simulink model "pos_control2_test"  (R2016b)
settings: Solver=ode3  StartTime=0.0  StopTime=30  FixedStep=0.0025  RelTol=1e-3
model workspace: external: MATLAB File /home/hywel/Simulink/2017_10_drone/para_pos.m (data not in the file)
undefined symbols (not defined in the file or in its folder): bool_pos, control_mode, def, par, par_input, par_pos, position_setpoint, v_control_mode
(part 1 of 2)
settings Model: Creator=root  LastModifiedBy=root
settings OptimizationCC: DefaultParameterBehavior=Inlined
settings DebuggingCC: ParameterTunabilityLossMsg=error
settings HardwareCC: ProdBitPerLong=64  ProdHWDeviceType=Intel->x86-64 (Linux 64)
settings RTWCC: SystemTargetFile=ert.tlc  TemplateMakefile=ert_default_tmf  Description=Embedded Coder  GenerateReport=on  IncludeHyperlinkInReport=on  LaunchReport=on  GenerateTraceInfo=on  GenerateTraceReport=on  GenerateTraceReportSl=on  GenerateTraceReportSf=on  GenerateTraceReportEml=on
settings CodeAppCC: ForceParamTrailComments=on  IgnoreCustomStorageClasses=off  OperatorAnnotations=on  SimulinkDataObjDesc=on  SFDataObjDesc=on  MATLABFcnDesc=on  InsertBlockDesc=on  MATLABSourceComments=on
settings ERTTargetCC: TargetLangStandard=C99 (ISO)  GenerateSampleERTMain=on  InlinedParameterPlacement=NonHierarchical  ERTCustomFileTemplate=example_file_process.tlc

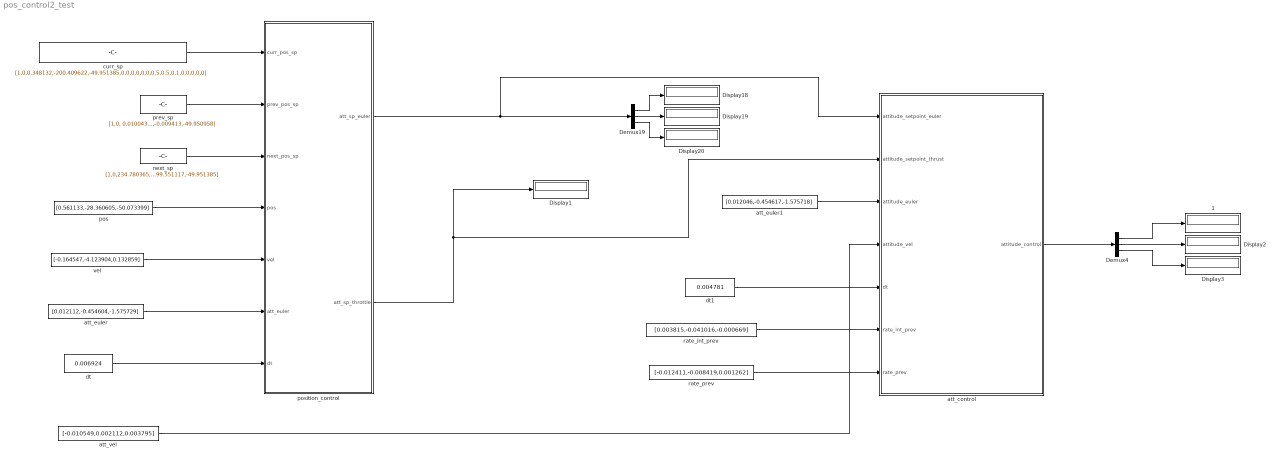
== system pos_control2_test ==
  1 : Display
  Demux19 : Demux  Outputs=3
  Demux4 : Demux  Outputs=3
  Display{1..3,18..20} (6 alike) : Display
  att_control : Subsystem
  att_euler : Constant  Value=[0.012112,-0.454604,-1.575729]
  att_euler1 : Constant  Value=[0.012046,-0.454617,-1.575718]
  att_vel : Constant  Value=[-0.010549,0.002112,0.003795]
  curr_sp : Constant  Value=[1,0,0.348132,-200.409622,-49.951385,0,0,0,0,0,0,0.5,0.5,0,1,0,0,0,0,0]
  dt : Constant  Value=0.006924
  dt1 : Constant  Value=0.004781
  next_sp : Constant  Value=[1,0,234.780365,-199.551117,-49.951385]
  pos : Constant  Value=[0.561133,-28.360605,-50.073399]
  position_control : Subsystem
  prev_sp : Constant  Value=[1,0, 0.010043,-0.009413,-49.950958]
  rate_int_prev : Constant  Value=[0.003815,-0.041016,-0.000669]
  rate_prev : Constant  Value=[-0.012411,-0.008419,0.001262]
  vel : Constant  Value=[-0.164547,-4.123904,0.132859]
  wires:
  pos/1 -> position_control/4(pos)
  vel/1 -> position_control/5(vel)
  curr_sp/1 -> position_control/1(curr_pos_sp)
  prev_sp/1 -> position_control/2(prev_pos_sp)
  next_sp/1 -> position_control/3(next_pos_sp)
  Demux19/2 -> Display19/1
  Demux19/3 -> Display20/1
  Demux19/1 -> Display18/1
  att_control/1(attitude_control) -> Demux4/1
  Demux4/2 -> Display2/1
  Demux4/1 -> 1/1
  Demux4/3 -> Display3/1
  att_euler/1 -> position_control/6(att_euler)
  att_vel/1 -> att_control/4(attitude_vel)
  dt/1 -> position_control/7(dt)
  rate_prev/1 -> att_control/7(rate_prev)
  rate_int_prev/1 -> att_control/6(rate_int_prev)
  dt1/1 -> att_control/5(dt)
  position_control/2(att_sp_throttle) -> att_control/2(attitude_setpoint_thrust), Display1/1
  position_control/1(att_sp_euler) -> att_control/1(attitude_setpoint_euler), Demux19/1
  att_euler1/1 -> att_control/3(attitude_euler)

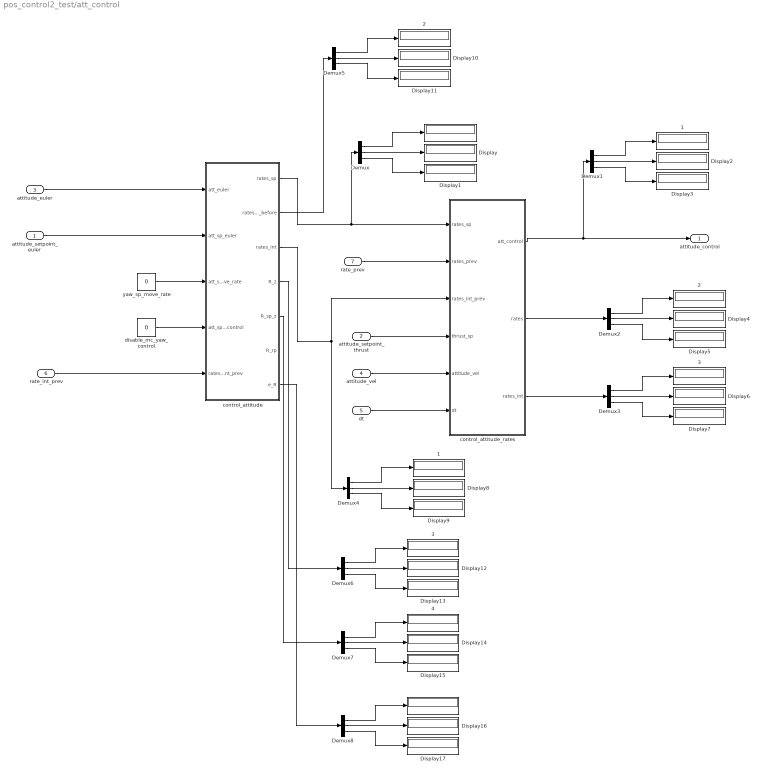
== system pos_control2_test/att_control ==
  attitude_setpoint_euler : Inport
  attitude_setpoint_thrust : Inport  Port=2
  attitude_euler : Inport  Port=3
  attitude_vel : Inport  Port=4
  dt : Inport  Port=5
  rate_int_prev : Inport  Port=6
  rate_prev : Inport  Port=7
   {,,1..4} (6 alike) : Display
  1 : Display
  2 : Display
  3 : Display
  Demux{,1..8} (9 alike) : Demux  Outputs=3
  Display{,1..17} (18 alike) : Display
  control_attitude : MATLAB Function  TreatAsAtomicUnit=on
  control_attitude_rates : MATLAB Function  TreatAsAtomicUnit=on
  disable_mc_yaw_control : Constant  Value=0
  yaw_sp_move_rate : Constant  Value=0
  attitude_control : Outport
  wires:
  yaw_sp_move_rate/1 -> control_attitude/3(att_sp_yaw_sp_move_rate)
  disable_mc_yaw_control/1 -> control_attitude/4(att_sp_disable_mc_yaw_control)
  control_attitude/1(rates_sp) -> Demux/1, control_attitude_rates/1(rates_sp)
  attitude_setpoint_euler/1 -> control_attitude/2(att_sp_euler)
  attitude_setpoint_thrust/1 -> control_attitude_rates/4(thrust_sp)
  attitude_euler/1 -> control_attitude/1(att_euler)
  attitude_vel/1 -> control_attitude_rates/5(attitude_vel)
  Demux/2 -> Display/1
  Demux/1 -> " "/1
  Demux/3 -> Display1/1
  control_attitude_rates/1(att_control) -> Demux1/1, attitude_control/1
  Demux1/2 -> Display2/1
  Demux1/1 -> 1/1
  Demux1/3 -> Display3/1
  control_attitude_rates/2(rates) -> Demux2/1
  Demux2/2 -> Display4/1
  Demux2/1 -> 2/1
  Demux2/3 -> Display5/1
  control_attitude_rates/3(rates_int) -> Demux3/1
  Demux3/2 -> Display6/1
  Demux3/1 -> 3/1
  Demux3/3 -> Display7/1
  dt/1 -> control_attitude_rates/6(dt)
  rate_int_prev/1 -> control_attitude/5(rates_int_prev)
  rate_prev/1 -> control_attitude_rates/2(rates_prev)
  control_attitude/3(rates_int) -> control_attitude_rates/3(rates_int_prev), Demux4/1
  Demux4/2 -> Display8/1
  Demux4/1 -> " 1"/1
  Demux4/3 -> Display9/1
  control_attitude/2(rates_sp_before) -> Demux5/1
  Demux5/2 -> Display10/1
  Demux5/1 -> " 2"/1
  Demux5/3 -> Display11/1
  control_attitude/4(R_z) -> Demux6/1
  Demux6/2 -> Display12/1
  Demux6/1 -> " 3"/1
  Demux6/3 -> Display13/1
  control_attitude/5(R_sp_z) -> Demux7/1
  Demux7/2 -> Display14/1
  Demux7/1 -> " 4"/1
  Demux7/3 -> Display15/1
  control_attitude/7(e_R) -> Demux8/1
  Demux8/2 -> Display16/1
  Demux8/1 -> " "/1
  Demux8/3 -> Display17/1

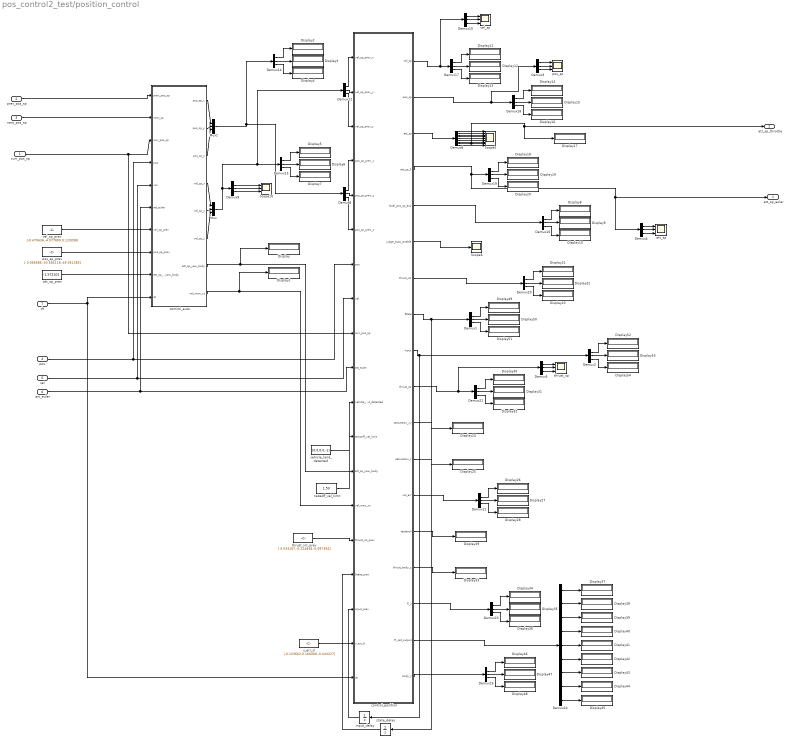
== system pos_control2_test/position_control ==
  curr_pos_sp : Inport
  prev_pos_sp : Inport  Port=2
  next_pos_sp : Inport  Port=3
  pos : Inport  Port=4
  vel : Inport  Port=5
  att_euler : Inport  Port=6
  dt : Inport  Port=7
  Demux{1..5,8..10,12,14..23,25} (20 alike) : Demux  Outputs=3
  Demux24 : Demux  Outputs=9
  Demux6 : Demux  Outputs=9
  Display{,1..54} (55 alike) : Display
  Mux : Mux  Inputs=3
  Mux1 : Mux  Inputs=3
  Scope10 : Scope  NumInputPorts=3
  Scope5 : Scope  NumInputPorts=9
  Scope6 : Scope
  att_sp : Scope  NumInputPorts=3
  att_sp_prev : Constant  Value=-1.572101
  control_auto : MATLAB Function  TreatAsAtomicUnit=on
  control_position : MATLAB Function  TreatAsAtomicUnit=on
  input_delay : UnitDelay  InitialCondition=[0,0,0]  SampleTime=-1
  pos_sp : Scope  NumInputPorts=3
  pos_sp_prev : Constant  Value=[ 0.066686,-33.584118,-49.951385]
  state_delay : UnitDelay  InitialCondition=[0,0,0]  SampleTime=-1
  takeoff_vel_limit : Constant  Value=1.53
  thrust_int_prev : Constant  Value=[ 0.034167,-0.224848,-0.087394]
  thrust_sp : Scope  NumInputPorts=3
  v_err_d : Constant  Value=[-0.123662,0.166068,-0.043227]
  vehicle_land_detected : Constant  Value=[0,0,0,0,-1]
  vel_sp : Scope  NumInputPorts=3
  vel_sp_prev : Constant  Value=[-0.470636,-4.977800,0.120098]
  att_sp_euler : Outport
  att_sp_throttle : Outport  Port=2
  wires:
  control_auto/7(att_sp_yaw_body) -> Display/1, control_position/13(att_sp_yaw_body)
  control_auto/8(vel_max_xy) -> Display1/1, control_position/14(vel_max_xy)
  takeoff_vel_limit/1 -> control_position/12(takeoff_vel_limit)
  vehicle_land_detected/1 -> control_position/11(vehicle_land_detected)
  next_pos_sp/1 -> control_auto/2(next_sp)
  prev_pos_sp/1 -> control_auto/1(prev_pos_sp)
  curr_pos_sp/1 -> control_auto/3(curr_pos_sp), control_position/9(curr_pos_sp)
  Demux6/1 -> Scope5/1
  Demux6/2 -> Scope5/2
  Demux6/3 -> Scope5/3
  control_position/3(att_sp) -> Demux6/1
  Demux6/4 -> Scope5/4
  Demux6/5 -> Scope5/5
  Demux6/6 -> Scope5/6
  Demux6/7 -> Scope5/7
  Demux6/9 -> Scope5/9
  control_position/5(local_pos_sp_acc) -> Demux16/1
  control_position/6(judge_auto_enable) -> Scope6/1
  Demux8/1 -> control_position/4(pos_sp_prev_x)
  Demux8/2 -> control_position/5(pos_sp_prev_y)
  Demux8/3 -> control_position/6(pos_sp_prev_z)
  Demux9/1 -> Scope10/1
  Demux9/2 -> Scope10/2
  Demux9/3 -> Scope10/3
  Demux12/1 -> control_position/1(vel_sp_prev_x)
  Demux12/2 -> control_position/2(vel_sp_prev_y)
  Demux12/3 -> control_position/3(vel_sp_prev_z)
  Demux14/2 -> Display3/1
  Demux14/3 -> Display4/1
  Demux14/1 -> Display2/1
  Demux15/2 -> Display6/1
  Demux15/3 -> Display7/1
  Demux15/1 -> Display5/1
  att_euler/1 -> control_position/10(att_euler), control_auto/6(att_euler)
  pos/1 -> control_auto/4(pos), control_position/7(pos)
  vel/1 -> control_position/8(vel), control_auto/5(vel)
  Demux16/2 -> Display9/1
  Demux16/3 -> Display10/1
  Demux16/1 -> Display8/1
  Demux17/2 -> Display12/1
  Demux17/3 -> Display13/1
  Demux17/1 -> Display11/1
  Demux18/2 -> Display15/1
  Demux18/3 -> Display16/1
  Demux18/1 -> Display14/1
  Demux19/2 -> Display19/1
  Demux19/3 -> Display20/1
  Demux19/1 -> Display18/1
  control_position/7(thrust_int) -> Demux20/1
  Demux20/2 -> Display22/1
  Demux20/3 -> Display23/1
  Demux20/1 -> Display21/1
  control_position/11(saturation_xy) -> Display24/1
  control_position/12(saturation_z) -> Display25/1
  control_position/13(vel_err) -> Demux21/1
  Demux21/2 -> Display27/1
  Demux21/3 -> Display28/1
  Demux21/1 -> Display26/1
  control_position/14(testbool) -> Display29/1
  Demux22/2 -> Display31/1
  Demux22/3 -> Display32/1
  Demux22/1 -> Display30/1
  control_position/15(thrust_body_z) -> Display33/1
  Demux23/2 -> Display35/1
  Demux23/3 -> Display36/1
  Demux23/1 -> Display34/1
  control_position/16(R_z) -> Demux23/1
  Demux24/1 -> Display37/1
  Demux24/2 -> Display38/1
  Demux24/3 -> Display39/1
  Demux24/4 -> Display40/1
  Demux24/5 -> Display41/1
  Demux24/6 -> Display42/1
  Demux24/7 -> Display43/1
  Demux24/8 -> Display44/1
  Demux24/9 -> Display45/1
  control_position/17(R_set_output) -> Demux24/1
  Demux25/2 -> Display47/1
  Demux25/3 -> Display48/1
  Demux25/1 -> Display46/1
  control_position/18(body_z) -> Demux25/1
  state_delay/1 -> control_position/16(State_prev)
  Demux1/2 -> Display50/1
  Demux1/3 -> Display51/1
  Demux1/1 -> Display49/1
  control_position/8(State) -> state_delay/1, Demux1/1
  input_delay/1 -> control_position/17(input_prev)
  Demux2/2 -> Display53/1
  Demux2/3 -> Display54/1
  Demux2/1 -> Display52/1
  control_position/9(input) -> input_delay/1, Demux2/1
  thrust_int_prev/1 -> control_position/15(thrust_int_prev)
  att_sp_prev/1 -> control_auto/9(att_sp_prev_yaw_body)
  vel_sp_prev/1 -> control_auto/7(vel_sp_prev)
  Demux6/8 -> Scope5/8, Display17/1, att_sp_throttle/1
  control_auto/5(vel_sp_y) -> Mux/2
  control_auto/4(vel_sp_x) -> Mux/1
  control_auto/6(vel_sp_z) -> Mux/3
  control_auto/2(pos_sp_y) -> Mux1/2
  control_auto/3(pos_sp_z) -> Mux1/3
  control_auto/1(pos_sp_x) -> Mux1/1
  control_position/1(vel_sp) -> Demux10/1, Demux17/1
  Demux10/1 -> vel_sp/1
  Demux10/2 -> vel_sp/2
  Demux10/3 -> vel_sp/3
  control_position/2(pos_sp) -> Demux3/1, Demux18/1
  Demux3/1 -> pos_sp/1
  Demux3/2 -> pos_sp/2
  Demux3/3 -> pos_sp/3
  control_position/4(att_sp_3) -> Demux4/1, att_sp_euler/1, Demux19/1
  Demux4/1 -> att_sp/1
  Demux4/2 -> att_sp/2
  Demux4/3 -> att_sp/3
  control_position/10(thrust_sp) -> Demux5/1, Demux22/1
  Demux5/1 -> thrust_sp/1
  Demux5/2 -> thrust_sp/2
  Demux5/3 -> thrust_sp/3
  v_err_d/1 -> control_position/18(v_err_d)
  dt/1 -> control_position/19(dt), control_auto/10(dt)
  Mux1/1 -> Demux8/1, Demux14/1
  pos_sp_prev/1 -> control_auto/8(pos_sp_prev)
  Mux/1 -> Demux12/1, Demux15/1, Demux9/1

== matlab function pos_control2_test/att_control/control_attitude ==
  data: att_euler input; att_sp_euler input; rates_sp output; rates_sp_before output; rates_int output; R_z output; R_sp_z output; R_rp output; att_sp_yaw_sp_move_rate input; att_sp_disable_mc_yaw_control input; rates_int_prev input; par parameter; v_control_mode parameter; e_R output
function [rates_sp,rates_sp_before,rates_int,R_z,R_sp_z,R_rp,e_R] = control_attitude(att_euler,att_sp_euler,att_sp_yaw_sp_move_rate,att_sp_disable_mc_yaw_control,rates_int_prev,par, v_control_mode)
%construct attitude setpoint rotation matrix
%get current rotation matrix from control state quaternions
rates_int = rates_int_prev;
I = diag([1,1,1]);
R_sp = euler_to_dcm(att_sp_euler);
R = euler_to_dcm(att_euler);
%R = q_to_dcm(v_att_q);
%try to move thrust vector shortest way, because yaw response is slower than roll/pitch
R_z = [R(1,3),R(2,3),R(3,3)]';
R_sp_z = [R_sp(1,3),R_sp(2,3),R_sp(3,3)]';

%axis and sin(angle) of desired rotation (indexes: 0=pitch, 1=roll, 2=yaw).
%This is for roll/pitch only (tilt), e_R(2) is 0
e_R = R'* cross(R_z,R_sp_z);

%calculate angle error
e_R_z_sin = norm(e_R);
e_R_z_cos = dot(R_z,R_sp_z);

%calculate rotation matrix after roll/pitch only rotation
R_rp = zeros(3);

if e_R_z_sin > 0.0
    %get axis-angle representation
    e_R_z_angle = atan(e_R_z_sin/e_R_z_cos);
    e_R_z_axis = e_R/e_R_z_sin;
    
    e_R = e_R_z_axis*e_R_z_angle;
    
    %cross product matrix for e_R_axis
    e_R_cp = zeros(3);
	e_R_cp(1, 2) = -e_R_z_axis(3);
	e_R_cp(1, 3) = e_R_z_axis(2);
	e_R_cp(2, 1) = e_R_z_axis(3);
	e_R_cp(2, 3) = -e_R_z_axis(1);
	e_R_cp(3, 1) = -e_R_z_axis(2);
	e_R_cp(3, 2) = e_R_z_axis(1);
    %rotation matrix for roll/pitch only rotation
    R_rp = R * (I + e_R_cp * e_R_z_sin + e_R_cp * e_R_cp * (1.0 - e_R_z_cos));
else
    %zero roll/pitch rotation 
    R_rp = R;
end

% R_rp and R_sp have the same Z axis, calculate yaw error 
R_sp_x = [R_sp(1, 1), R_sp(2, 1), R_sp(3, 1)]';
R_rp_x = [R_rp(1, 1), R_rp(2, 1), R_rp(3, 1)]';
    
%  calculate the weight for yaw control
%  Make the weight depend on the tilt angle error: the higher the error of roll and/or pitch, the lower
%  the weight that we use to control the yaw. This gives precedence to roll & pitch correction.
%  The weight is 1 if there is no tilt error.
yaw_w = e_R_z_cos*e_R_z_cos;

e_R(3) = atan(dot(cross(R_rp_x,R_sp_x),R_sp_z)/dot(R_rp_x,R_sp_x)) * yaw_w;
if e_R_z_cos<0.0
    q_error = dcm_to_q(R'*R_sp);
    if q_error >= 0.0
        e_R_d = [q_error(2),q_error(3),q_error(4)]'*2;
    else
        e_R_d = [-q_error(2),-q_error(3),-q_error(4)]'*2;
    end
    % use fusion of Z axis based rotation and direct rotation
    direct_w = e_R_z_cos * e_R_z_cos * yaw_w;
    e_R = e_R * (1.0 - direct_w) + e_R_d * direct_w;
end

% calculate angular rates setpoint
rates_sp = [par.att_p(1)*e_R(1),par.att_p(2)*e_R(2),par.att_p(3)*e_R(3)]';
% Feed forward the yaw setpoint rate. We need to transform the yaw from world into body frame.
% The following is a simplification of:
yaw_feedforward_rate = [R(3, 1), R(3, 2), R(3, 3)]';
yaw_feedforward_rate = yaw_feedforward_rate * att_sp_yaw_sp_move_rate * par.yaw_ff;

yaw_feedforward_rate(3) = yaw_feedforward_rate(3) * yaw_w;
rates_sp = rates_sp + yaw_feedforward_rate;

rates_sp_before = rates_sp;

% limit rates
for i = 1:2
    if (v_control_mode.flag_control_velocity_enabled || v_control_mode.flag_control_auto_enabled) && ~v_control_mode.flag_control_manual_enabled
        rates_sp(i) = constrain(rates_sp(i), -par.auto_rate_max(i), par.auto_rate_max(i));
    else
        rates_sp(i) = constrain(rates_sp(i), -par.mc_rate_max(i), par.mc_rate_max(i));
    end
end
        
if (v_control_mode.flag_control_velocity_enabled || v_control_mode.flag_control_auto_enabled) && att_sp_disable_mc_yaw_control == true && ~v_control_mode.flag_control_manual_enabled
    wv_yaw_rate_max = par.auto_rate_max(3) * par.vtol_wv_yaw_rate_scale;
    rates_sp(3) = constrain(rates_sp(3), -wv_yaw_rate_max, wv_yaw_rate_max);
	%prevent integrator winding up in weathervane mode
	rates_int(3) = 0.0;
end

== matlab function pos_control2_test/att_control/control_attitude_rates ==
  data: rates_sp input; rates_prev input; rates_int_prev input; thrust_sp input; attitude_vel input; att_control output; par parameter; rates output; rates_int output; def parameter; dt input
function [att_control,rates,rates_int] = control_attitude_rates(rates_sp, rates_prev,rates_int_prev ,thrust_sp, attitude_vel, par, def, dt)

rates_int = rates_int_prev;
%/* reset integral if disarmed */
%if (!_armed.armed || !_vehicle_status.is_rotary_wing) {
%rates_int = zero(1,3);
%}
%get the raw gyro data and correct for thermal errors

rates = zeros(3,1);

rates(1) = attitude_vel(1);
rates(2) = attitude_vel(2);
rates(3) = attitude_vel(3);
%rates(1) = (sensor_angular_vel(1) - sensor_offset(1)) * sensor_scale(1);
%rates(2) = (sensor_angular_vel(2) - sensor_offset(2)) * sensor_scale(2); 
%rates(3) = (sensor_angular_vel(3) - sensor_offset(3)) * sensor_scale(3); 

%rotate corrected measurements from sensor to body frame
%rates = par.board_rotation*rates;
%correct for in-run bias errors
%rates(1) = rates(1)-sensor_gyro_bias(1);
%rates(2) = rates(2)-sensor_gyro_bias(2);
%rates(3) = rates(3)-sensor_gyro_bias(3);

pid_p = pid_attenuations(par.tpa_breakpoint_p,par.tpa_rate_p,thrust_sp,def);
rates_p_scaled = [par.rate_p(1)*pid_p(1),par.rate_p(2)*pid_p(2),par.rate_p(3)*pid_p(3)]';

pid_d = pid_attenuations(par.tpa_breakpoint_d,par.tpa_rate_d,thrust_sp,def);
rates_d_scaled = [par.rate_d(1)*pid_d(1),par.rate_d(2)*pid_d(2),par.rate_d(3)*pid_d(3)]';

% angular rates error
rates_err = rates_sp - rates;

att_control = rates_p_scaled.*rates_err + rates_int + rates_d_scaled.*(rates_prev - rates)/dt + par.rate_ff.*rates_sp;

% update integral only if motors are providing enough thrust to be effective
if thrust_sp > def.MIN_TAKEOFF_THRUST
    for i = def.AXIS_INDEX_ROLL:def.AXIS_COUNT
        %Check for positive control saturation
        %todo
        %positive_saturation =((i == def.AXIS_INDEX_ROLL) && saturation_status.flags.roll_pos) ||((i == def.AXIS_INDEX_PITCH) && saturation_status.flags.pitch_pos) ||((i == def.AXIS_INDEX_YAW) && saturation_status.flags.yaw_pos);
        positive_saturation = 0;
		%Check for negative control saturation
        %negative_saturation =((i == def.AXIS_INDEX_ROLL) && saturation_status.flags.roll_neg) ||((i == def.AXIS_INDEX_PITCH) && saturation_status.flags.pitch_neg) ||((i == def.AXIS_INDEX_YAW) && saturation_status.flags.yaw_neg);
        negative_saturation = 0;
		%prevent further positive control saturation
        if (positive_saturation) 
            rates_err(i) = min(rates_err(i), 0.0);
        end

		%prevent further negative control saturation
        if (negative_saturation) 
            rates_err(i) = max(rates_err(i), 0.0);
        end
		
		%Perform the integration using a first order method and do not propaate the result if out of range or invalid
        rate_i = rates_int(i) + par.rate_i(i) * rates_err(i) * dt;
        
        if (rate_i > -par.rate_int_lim(i) && rate_i < par.rate_int_lim(i))
            rates_int(i) = rate_i;
        end
    end
end

%explicitly limit the integrator state */
for i = def.AXIS_INDEX_ROLL:def.AXIS_COUNT
    rates_int(i) = constrain(rates_int(i), -par.rate_int_lim(i), par.rate_int_lim(i));
end

== matlab function pos_control2_test/position_control/control_auto ==
  data: prev_pos_sp input; next_sp input; curr_pos_sp input; pos input; vel input; att_euler input; vel_sp_prev input; pos_sp_prev input; att_sp_prev_yaw_body input; pos_sp_x output; pos_sp_y output; pos_sp_z output; vel_sp_x output; vel_sp_y output; vel_sp_z output; att_sp_yaw_body output; vel_max_xy output; def parameter; bool_pos parameter; position_setpoint parameter; par_pos parameter; dt input
function [pos_sp_x,pos_sp_y,pos_sp_z,vel_sp_x,vel_sp_y,vel_sp_z,att_sp_yaw_body,vel_max_xy] = control_auto(prev_pos_sp,next_sp,curr_pos_sp,pos,vel,att_euler,vel_sp_prev,pos_sp_prev,att_sp_prev_yaw_body,def, bool_pos, position_setpoint,par_pos, dt)
%curr_pos_sp(valid,type,x,y,z,vx,vy,vz,ax,ay,az,yaw,yawspeed,cruising_speed,position_valid,velocity_valid,acceleration_valid,yaw_valid,yawspeed_valid,cruising_valid)
%[1,0,10,10,10,0.1,0.1,0.1,0,0,0,1,0.1,0,1,1,0,1,0,0]
%prev_sp,next_sp [valid,type,x,y,z]
vel_max_xy = par_pos.vel_max_xy;
pos_sp = zeros(3,1);
pos_sp = pos_sp_prev;
vel_sp = zeros(3,1);
vel_sp = vel_sp_prev;
yaw = att_euler(3);
att_sp_yaw_body = att_sp_prev_yaw_body;
% reset position setpoint on AUTO mode activation or if we are not in MC mode */
if ~bool_pos.mode_auto
    bool_pos.mode_auto = 1;
    %set _triplet_lat_lon_finite true once switch to AUTO(e.g. LAND)
    bool_pos.triplet_lat_lon_finite = 1;

end

bool_pos.reset_pos_sp = 1;
bool_pos.reset_alt_sp = 1;

% Always check reset state of altitude and position control flags in auto
if (bool_pos.reset_pos_sp)
   bool_pos.reset_pos_sp = 0;
   pos_sp(1) = pos(1);
   pos_sp(2) = pos(2);
end

if (bool_pos.reset_alt_sp)
    bool_pos.reset_alt_sp = 0;
    pos_sp(3) = pos(3);
end

% init bool and vector
%bool
current_setpoint_valid = 0;
previous_setpoint_valid = 0;
next_setpoint_valid = 0;
triplet_updated = 0;

if (curr_pos_sp(1))

    %math::Vector<3> 
    %curr_pos_sp = _curr_pos_sp;

    %only project setpoints if they are finite, else use current position
     
    %if (PX4_ISFINITE(_pos_sp_triplet.current.lat) &&
       % PX4_ISFINITE(_pos_sp_triplet.current.lon)) {
        % project setpoint to local frame */
        %map_projection_project(&_ref_pos, _pos_sp_triplet.current.lat, _pos_sp_triplet.current.lon,&curr_pos_sp.data[0], &curr_pos_sp.data[1]);

        %_triplet_lat_lon_finite = true;

    %} else { % use current position if NAN -> e.g. land
       % if (_triplet_lat_lon_finite) {
        %    curr_pos_sp.data[0] = _pos(0);
         %   curr_pos_sp.data[1] = _pos(1);
       %     _triplet_lat_lon_finite = false;
        %}
    % only project setpoints if they are finite, else use current position
    % todo ref_alt
    %if (PX4_ISFINITE(_pos_sp_triplet.current.alt)) {
        %curr_pos_sp(5) = -(_pos_sp_triplet.current.alt - _ref_alt);
   % }
    % sanity check */
    if (isreal(curr_pos_sp(3)) && isreal(curr_pos_sp(4)) && isreal(curr_pos_sp(5)))
        current_setpoint_valid = 1;
    end

    % check if triplets have been updated
    % note: we only can look at xy since navigator applies slewrate to z */
    %float  diff;
    %if (_triplet_lat_lon_finite) {
       % diff = matrix::Vector2f((_curr_pos_sp(0) - curr_pos_sp(0)), (_curr_pos_sp(1) - curr_pos_sp(1))).length();
    %} else {
       % diff = fabsf(_curr_pos_sp(2) - curr_pos_sp(2));
    %}
    %if (diff > FLT_EPSILON) {
    %    triplet_updated = true;
    %}
    % we need to update _curr_pos_sp always since navigator applies slew rate on z */
    %_curr_pos_sp = curr_pos_sp;
end

if (prev_pos_sp(1))
    if (isreal(prev_pos_sp(3)) && isreal(prev_pos_sp(4)) && isreal(prev_pos_sp(5)))
        %_prev_pos_sp = prev_sp;
        previous_setpoint_valid = 1;
    end
end

% set previous setpoint to current position if no previous setpoint available */
if (~previous_setpoint_valid && triplet_updated)
    prev_pos_sp(3) = pos(1);
    prev_pos_sp(4) = pos(2);
    prev_pos_sp(5) = pos(3);
    previous_setpoint_valid = 1; % currrently not necessary to set to true since not used*/
end

if (next_sp(1))
    if (isreal(next_sp(3)) && isreal(next_sp(4)) && isreal(next_sp(5)))
        next_setpoint_valid = 1;
    end
end

%change curr_pos_sp, prev_pos_sp, next_sp
%todo
%current_setpoint_valid = 1;

%create new _pos_sp from triplets
if (current_setpoint_valid && curr_pos_sp(2) ~= position_setpoint.SETPOINT_TYPE_IDLE)
    % update yaw setpoint if needed
    if (curr_pos_sp(19) && position_setpoint.SETPOINT_TYPE_FOLLOW_TARGET)
        att_sp_yaw_body = att_sp_prev_yaw_body + curr_pos_sp(13)*dt;
    elseif (curr_pos_sp(18))
        att_sp_yaw_body = curr_pos_sp(12);
    end
    
    yaw_diff = wrap_pi(att_sp_yaw_body - yaw);
    
    % only follow previous-current-line for specific triplet type
    
    if  (curr_pos_sp(2) == position_setpoint.SETPOINT_TYPE_POSITION  ||curr_pos_sp(2) == position_setpoint.SETPOINT_TYPE_LOITER ||curr_pos_sp(2) == position_setpoint.SETPOINT_TYPE_FOLLOW_TARGET)
        %by default use current setpoint as is
        pos_sp = [curr_pos_sp(3);curr_pos_sp(4);curr_pos_sp(5)];
        
        %Z-DIRECTION
        
        % get various distances
        
		total_dist_z = abs(curr_pos_sp(5) - prev_pos_sp(5));
		dist_to_prev_z = abs(pos(3) - prev_pos_sp(5));
		dist_to_current_z = abs(curr_pos_sp(5) - pos(3));
        
        %  if pos_sp has not reached target setpoint (=curr_pos_sp(2)),
		%  then compute setpoint depending on vel_max
        if (total_dist_z >  def.SIGMA_NORM) && (abs(pos_sp(3) - curr_pos_sp(5)) > def.SIGMA_NORM)
            %%% ???
            flying_upward = (curr_pos_sp(5) < pos(3));
            
            % final_vel_z is the max velocity which depends on the distance of total_dist_z
			% with default params.vel_max_up/down
            if flying_upward
                final_vel_z = par_pos.vel_max_up;
            else
                final_vel_z = par_pos.vel_max_down;
            end
            % target threshold defines the distance to _curr_pos_sp(2) at which
			% the vehicle starts to slow down to approach the target smoothly
            target_threshold_z = final_vel_z * 1.5;
            % if the total distance in z is NOT 2x distance of target_threshold, we
			% will need to adjust the final_vel_z
			is_2_target_threshold_z = total_dist_z >= 2.0 * target_threshold_z;
			
            slope = (final_vel_z) / (target_threshold_z); % defines the the acceleration when slowing down */
			min_vel_z = 0.2; % minimum velocity: this is needed since estimation is not perfect
            
            if (~is_2_target_threshold_z)
				% adjust final_vel_z since we are already very close
				% to current and therefore it is not necessary to accelerate
				% up to full speed (=final_vel_z)
				target_threshold_z = total_dist_z * 0.5;
				%get the velocity at target_threshold_z */
				final_vel_z_tmp = slope * (target_threshold_z) + min_vel_z;

				%make sure that final_vel_z is never smaller than 0.5 of the default final_vel_z
				%this is mainly done because the estimation in z is not perfect and therefore
				%it is necessary to have a minimum speed

				final_vel_z = constrain(final_vel_z_tmp, final_vel_z * 0.5, final_vel_z);
            end

			vel_sp_z = final_vel_z;

			%we want to slow down */
            if (dist_to_current_z < target_threshold_z) 
                vel_sp_z = slope * dist_to_current_z + min_vel_z;
            elseif (dist_to_prev_z < target_threshold_z)
				%we want to accelerate */

				acc_z = (vel_sp_z - abs(vel_sp(3))) / dt;
                if flying_upward
                    acc_max = par_pos.acceleration_z_max_up * 0.5;
                else
                    acc_max = par_pos.acceleration_z_max_down * 0.5;
                end
                
                if (acc_z > acc_max)
                    vel_sp_z = par_pos.acceleration_z_max_up * dt + abs(vel_sp(3));
                end

            end

			%if we already close to current, then just take over the velocity that
			%we would have computed if going directly to the current setpoint
            if (vel_sp_z >= (dist_to_current_z * par_pos.pos_p(3)))
				vel_sp_z = dist_to_current_z * par_pos.pos_p(3);
            end

			% make sure vel_sp_z is always positive */
			vel_sp_z = constrain(vel_sp_z, 0.0, final_vel_z);
			% get the sign of vel_sp_z */
            if flying_upward
                vel_sp_z = -vel_sp_z ;
            %else
               % vel_sp_z = vel_sp_z;
            end
			% compute pos_sp(2) */
			pos_sp(3) = pos(3) + vel_sp_z / par_pos.pos_p(3);
        end
        
        
        % XY-DIRECTION


		% line from previous to current and from pos to current */
        vec_prev_to_current = [(curr_pos_sp(3) - prev_pos_sp(3)); (curr_pos_sp(4) - prev_pos_sp(4))];
        vec_pos_to_current = [(curr_pos_sp(3) - pos(1)); (curr_pos_sp(4) - pos(2))];


		% check if we just want to stay at current position */
		pos_sp_diff = [(curr_pos_sp(3) - pos_sp(1)); (curr_pos_sp(4) - pos_sp(2))];
		% bool
        stay_at_current_pos = (curr_pos_sp(2) == position_setpoint.SETPOINT_TYPE_LOITER || ~next_setpoint_valid) && (normest(pos_sp_diff) < def.SIGMA_NORM);

        % only follow line if previous to current has a minimum distance */

		% only follow line if previous to current has a minimum distance */
        if ((normest(vec_prev_to_current)  > par_pos.nav_rad ) && ~stay_at_current_pos) 

			% normalize prev-current line (always > nav_rad) */
			unit_prev_to_current = vec_prev_to_current/normest(vec_prev_to_current);

			% unit vector from current to next */
			unit_current_to_next = [0.0; 0.0];
            
            if (next_setpoint_valid) 
					unit_current_to_next = [(next_sp(3) - pos_sp(1)); (next_sp(4) - pos_sp(2))];
                    if normest(unit_current_to_next) > def.SIGMA_NORM
                        unit_current_to_next = unit_current_to_next/normest(unit_current_to_next);
                    %else
                        %unit_current_to_next;
                    end
            end

			% point on line closest to pos */
			closest_point = [prev_pos_sp(3); prev_pos_sp(4)] + unit_prev_to_current * ([(pos(1) - prev_pos_sp(3)), (pos(2) - prev_pos_sp(4))] * unit_prev_to_current);

			vec_closest_to_current = [(curr_pos_sp(3) - closest_point(1)); (curr_pos_sp(4) - closest_point(2))];

			% compute vector from position-current and previous-position */
			vec_prev_to_pos = [(pos(1) - prev_pos_sp(3)); (pos(2) - prev_pos_sp(4))];

			% current velocity along track */
			vel_sp_along_track_prev = dot([vel_sp(1); vel_sp(2)], unit_prev_to_current);

			% distance to target when brake should occur */
            if (curr_pos_sp(20) == 1 && ~(curr_pos_sp(14) < 0.0))
                %float
                get_cruising_speed_xy = curr_pos_sp(14);
            else
                get_cruising_speed_xy = par_pos.vel_cruise_xy;
            end
            
			target_threshold_xy = 1.5 * get_cruising_speed_xy;

            %bool
			close_to_current = normest(vec_pos_to_current) < target_threshold_xy;
            %bool
			close_to_prev = (normest(vec_prev_to_pos) < target_threshold_xy) && (normest(vec_prev_to_pos) < normest(vec_pos_to_current));

			% indicates if we are at least half the distance from previous to current close to previous */
			%bool
            is_2_target_threshold = normest(vec_prev_to_current) >= 2.0 * target_threshold_xy;

			% check if the current setpoint is behind */
			%bool
            current_behind = dot((vec_pos_to_current * -1.0), unit_prev_to_current) > 0.0;

			% check if the previous is in front */
			%bool 
            previous_in_front = dot(vec_prev_to_pos, unit_prev_to_current) < 0.0;

			% default velocity along line prev-current */
			%float 
            vel_sp_along_track = get_cruising_speed_xy;

		    %compute velocity setpoint along track

			% only go directly to previous setpoint if more than 5m away and previous in front*/
            if (previous_in_front && (normest(vec_prev_to_pos) > 5.0))
                % just use the default velocity along track */
                vel_sp_along_track = normest(vec_prev_to_pos) * par_pos.pos_p(1);
                if (vel_sp_along_track > get_cruising_speed_xy) 
                    vel_sp_along_track = get_cruising_speed_xy;
                end

            elseif (current_behind)
				% go directly to current setpoint */
				vel_sp_along_track = normest(vec_pos_to_current) * par_pos.pos_p(1);
                if (vel_sp_along_track < get_cruising_speed_xy)
                    %vel_sp_along_track = vel_sp_along_track;
                else
                    vel_sp_along_track = get_cruising_speed_xy;
                end

            elseif (close_to_prev)
				% accelerate from previous setpoint towards current setpoint */

				% we are close to previous and current setpoint
				% we first compute the start velocity when close to current septoint and use
				% this velocity as final velocity when transition occurs from acceleration to deceleration.
				% This ensures smooth transition */
				%float 
                final_cruise_speed = get_cruising_speed_xy;
                
                if (~is_2_target_threshold)
                    % set target threshold to half dist pre-current */
                    %float
                    target_threshold_tmp = target_threshold_xy;
                    target_threshold_xy = normest(vec_prev_to_current) * 0.5;
                    if ((target_threshold_xy - par_pos.nav_rad ) < def.SIGMA_NORM)
                        target_threshold_xy = par_pos.nav_rad ;
                    end

					% velocity close to current setpoint with default zero if no next setpoint is available */
					%float 
                    vel_close = 0.0;
					%float 
                    acceptance_radius = 0.0;

					% we want to pass and need to compute the desired velocity close to current setpoint */
                    if (next_setpoint_valid &&  ~(curr_pos_sp(2) == position_setpoint.SETPOINT_TYPE_LOITER))
                        % get velocity close to current that depends on angle between prev-current and current-next line */
                        vel_close = get_vel_close(get_cruising_speed_xy,unit_prev_to_current, unit_current_to_next);
                        acceptance_radius = par_pos.nav_rad;
                    end

					% compute velocity at transition where vehicle switches from acceleration to deceleration */
                    if ((target_threshold_tmp - acceptance_radius) < def.SIGMA_NORM)
                        final_cruise_speed = vel_close;

                    else
                        %float 
                        slope = (get_cruising_speed_xy - vel_close) / (target_threshold_tmp - acceptance_radius);
                        final_cruise_speed = slope  * (target_threshold_xy - acceptance_radius) + vel_close;
                        if final_cruise_speed > vel_close
                            %final_cruise_speed = final_cruise_speed;
                        else
                            final_cruise_speed = vel_close;
                        end
                    end
                end

				% make sure final cruise speed is larger than 0*/
                if final_cruise_speed > def.SIGMA_NORM
                    %final_cruise_speed = final_cruise_speed;
                else
                    final_cruise_speed = def.SIGMA_NORM;
                end
                
				vel_sp_along_track = final_cruise_speed;

				% we want to accelerate not too fast
				% TODO: change the name acceleration_hor_man to something that can
				% be used by auto and manual */
				
                %float 
                acc_track = (final_cruise_speed - vel_sp_along_track_prev) / dt;

				% if yaw offset is large, only accelerate with 0.5m/s^2 */
				
                %float 
                if (abs(yaw_diff) >  par_pos.mis_yaw_error *def.M_PI_F/180)
                    acc = 0.5;
                else
                    acc = par_pos.acceleration_hor;
                end
                
                if (acc_track > acc)
                    vel_sp_along_track = acc * dt + vel_sp_along_track_prev;
                end

				% enforce minimum cruise speed */
				vel_sp_along_track  = constrain(vel_sp_along_track, def.SIGMA_NORM, final_cruise_speed);
                
            elseif (close_to_current)
				% slow down when close to current setpoint */

				% check if altidue is within acceptance radius */
                %bool 
                if dist_to_current_z < par_pos.nav_rad
                    reached_altitude = 1;
                else
                    reached_altitude = 0;
                end
                
                if (reached_altitude && next_setpoint_valid && ~(curr_pos_sp(2) == position_setpoint.SETPOINT_TYPE_LOITER))
                    % since we have a next setpoint use the angle prev-current-next to compute velocity setpoint limit */

					% get velocity close to current that depends on angle between prev-current and current-next line */
                    %float 
                    vel_close = get_vel_close(get_cruising_speed_xy,unit_prev_to_current, unit_current_to_next);

					% compute velocity along line which depends on distance to current setpoint */
                    if (normest(vec_closest_to_current) < par_pos.nav_rad)
						vel_sp_along_track = vel_close;
                    else
                        if (target_threshold_xy - par_pos.nav_rad < def.SIGMA_NORM)
							vel_sp_along_track = vel_close;
                        else
							%float 
                            slope = (get_cruising_speed_xy - vel_close) / (target_threshold_xy - par_pos.nav_rad) ;
							vel_sp_along_track = slope  * (normest(vec_closest_to_current) - par_pos.nav_rad) + vel_close;
                        end
                    end

					% since we want to slow down take over previous velocity setpoint along track if it was lower */
                    if ((vel_sp_along_track_prev < vel_sp_along_track) && (vel_sp_along_track * vel_sp_along_track_prev > 0.0))
							vel_sp_along_track = vel_sp_along_track_prev;
                    end

					% if we are close to target and the previous velocity setpoints was smaller than
					% vel_sp_along_track, then take over the previous one
					% this ensures smoothness since we anyway want to slow down
                    if ((vel_sp_along_track_prev < vel_sp_along_track) && (vel_sp_along_track * vel_sp_along_track_prev > 0.0) && (vel_sp_along_track_prev > vel_close)) 
                        vel_sp_along_track = vel_sp_along_track_prev;
                    end

					% make sure that vel_sp_along track is at least min */
                    if vel_sp_along_track < vel_close
                        vel_sp_along_track = vel_close;
                    end
				else 

					% we want to stop at current setpoint */
					%float 
                    slope = (get_cruising_speed_xy)  / target_threshold_xy;
					vel_sp_along_track =  slope * (normest(vec_closest_to_current));

					% since we want to slow down take over previous velocity setpoint along track if it was lower but ensure its not zero */
                    if ((vel_sp_along_track_prev < vel_sp_along_track) && (vel_sp_along_track * vel_sp_along_track_prev > 0.0) && (vel_sp_along_track_prev > 0.5)) 
                        vel_sp_along_track = vel_sp_along_track_prev;
                    end
                end
            end
            
            % compute velocity orthogonal to prev-current-line to position*/
            %matrix::Vector2f 
            vec_pos_to_closest = closest_point - [pos(1); pos(2)];
            %float 
            vel_sp_orthogonal = normest(vec_pos_to_closest) * par_pos.pos_p(1);

			% compute the cruise speed from velocity along line and orthogonal velocity setpoint */
            %float 
            cruise_sp_mag = sqrt(vel_sp_orthogonal * vel_sp_orthogonal + vel_sp_along_track * vel_sp_along_track);

			% sanity check *
            if ~isreal(cruise_sp_mag)
                cruise_sp_mag = vel_sp_orthogonal;
            end

			% orthogonal velocity setpoint is smaller than cruise speed */
            if (vel_sp_orthogonal < get_cruising_speed_xy && ~current_behind)

                % we need to limit vel_sp_along_track such that cruise speed  is never exceeded but still can keep velocity orthogonal to track */
                if (cruise_sp_mag > get_cruising_speed_xy)
					vel_sp_along_track = sqrt(get_cruising_speed_xy * get_cruising_speed_xy - vel_sp_orthogonal * vel_sp_orthogonal);
                end

				pos_sp(1) = closest_point(1) + unit_prev_to_current(1) * vel_sp_along_track / par_pos.pos_p(1);
				pos_sp(2) = closest_point(2) + unit_prev_to_current(2) * vel_sp_along_track / par_pos.pos_p(2);
            elseif (current_behind)
                % current is behind */
                if (normest(vec_pos_to_current)  > 0.01) 
                    pos_sp(1) = pos(1) + vec_pos_to_current(1) / normest(vec_pos_to_current) * vel_sp_along_track / par_pos.pos_p(1);
                    pos_sp(2) = pos(2) + vec_pos_to_current(2) / normest(vec_pos_to_current) * vel_sp_along_track / par_pos.pos_p(2);

                else
                    pos_sp(1) = curr_pos_sp(3);
                    pos_sp(2) = curr_pos_sp(4);
                end
            else
                % we are more than cruise_speed away from track */
                % if previous is in front just go directly to previous point */
                if (previous_in_front)
                    vec_pos_to_closest(1) = prev_pos_sp(3) - pos(1);
                    vec_pos_to_closest(2) = prev_pos_sp(4) - pos(2);
                end
                
                % make sure that we never exceed maximum cruise speed */
                %float 
                cruise_sp = normest(vec_pos_to_closest) * par_pos.pos_p(1);
                
                if (cruise_sp > get_cruising_speed_xy)
                    cruise_sp = get_cruising_speed_xy;
                end
                
                % sanity check: don't divide by zero */
                if (normest(vec_pos_to_closest) > def.SIGMA_NORM)
                    pos_sp(1) = pos(1) + vec_pos_to_closest(1) / normest(vec_pos_to_closest) * cruise_sp / par_pos.pos_p(1);
                    pos_sp(2) = pos(2) + vec_pos_to_closest(2) / normest(vec_pos_to_closest) * cruise_sp / par_pos.pos_p(2);
                else
                    pos_sp(1) = closest_point(1);
                    pos_sp(2) = closest_point(2);
                end
            end
        end
        %pos_sp = pos_sp;
    elseif (curr_pos_sp(2) == position_setpoint.SETPOINT_TYPE_VELOCITY)
        if (curr_pos_sp(20) == 1 && ~(curr_pos_sp(14) < 0.0))
            %float
            get_cruising_speed_xy = curr_pos_sp(14);
        else
            get_cruising_speed_xy = par_pos.vel_cruise_xy;
        end

        %float 
        vel_xy_mag = sqrt(vel(1) * vel(1) + vel(2) * vel(2));

        if (vel_xy_mag > def.SIGMA_NORM)
            vel_sp(1) = vel(1) / vel_xy_mag * get_cruising_speed_xy;
            vel_sp(2) = vel(2) / vel_xy_mag * get_cruising_speed_xy;

        else
            % TODO: we should go in the direction we are heading
            % if current velocity is zero
            %
            vel_sp(1) = 0.0;
            vel_sp(2) = 0.0;
        end

        bool_pos.run_pos_control = 0;

    else
        % just go to the target point */;
        pos_sp(1) = curr_pos_sp(3);
        pos_sp(2) = curr_pos_sp(4);
        pos_sp(3) = curr_pos_sp(5);
        
        if (curr_pos_sp(20) == 1 && ~(curr_pos_sp(14) < 0.0))
            %float
            get_cruising_speed_xy = curr_pos_sp(14);
        else
            get_cruising_speed_xy = par_pos.vel_cruise_xy;
        end

        % set max velocity to cruise */
        vel_max_xy = get_cruising_speed_xy;
    end
    

    % sanity check */
    if (~(isreal(pos_sp(1)) && isreal(pos_sp(2)) && isreal(pos_sp(3))))

        %warn_rate_limited("Auto: Position setpoint not finite");
        pos_sp(1) = curr_pos_sp(3);
        pos_sp(2) = curr_pos_sp(4);
        pos_sp(3) = curr_pos_sp(5);
    end
    
    % if we're already near the current takeoff setpoint don't reset in case we switch back to posctl.
    % this makes the takeoff finish smoothly.
	% todo
else
    vel_sp = zeros(3,1);
    bool_pos.run_pos_control = 0;
	bool_pos.run_alt_control = 0;
end


pos_sp_x = pos_sp(1);
pos_sp_y = pos_sp(2);
pos_sp_z = pos_sp(3);
vel_sp_x = vel_sp(1);
vel_sp_y = vel_sp(2);
vel_sp_z = vel_sp(3);
